simulink model "modeloLineales"  (R2022a)
settings: Solver=VariableStepAuto  StartTime=0.0  StopTime=300  FixedStep=6  RelTol=1e-3
model workspace (MAT data in the model file):
  ca = 0.001
  cb = 0.001
  ea = 0.001
  eb = 0.001
  pa = 2
  pb = 2
  u = 0.001
  v = 3
settings Model: Creator=Asus  LastModifiedBy=Abelino
settings DataIOCC: SaveFormat=Array  OutputTimes=tout

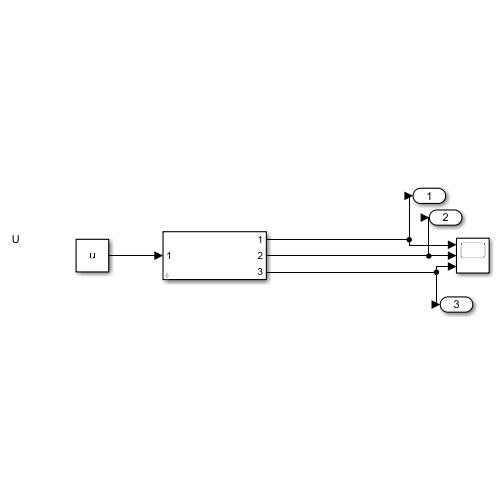
[thumbnail: Simulink's stored preview of the top-level diagram]
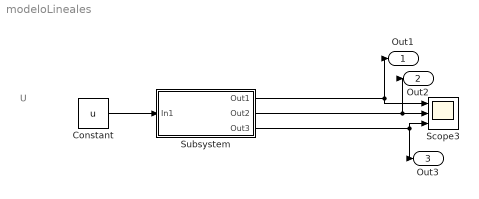
== system modeloLineales ==
  note: U
  Constant : Constant  Value=u
  Scope3 : Scope  NumInputPorts=3
  Subsystem : Subsystem  mask{ea=ea, eb=eb, ca=ca, cb=cb, pa=pa, pb=pb, v=v}
      mask prompts: ea "Tasa de extinción competidor A"; eb "Tasa de extinción del competidor B"; ca "Tasa de colonización del competidor A"; cb "Tasa de colonización del competidor B"; pa "Condición inicial x1"; pb "Condicion inicial x2"; v "Condicion inicial x3"
  Out1 : Outport
  Out2 : Outport  Port=2
  Out3 : Outport  Port=3
  wires:
  Subsystem/2(Out2) -> Out2/1, Scope3/2
  Subsystem/3(Out3) -> Scope3/3, Out3/1
  Subsystem/1(Out1) -> Scope3/1, Out1/1
  Constant/1 -> Subsystem/1(In1)

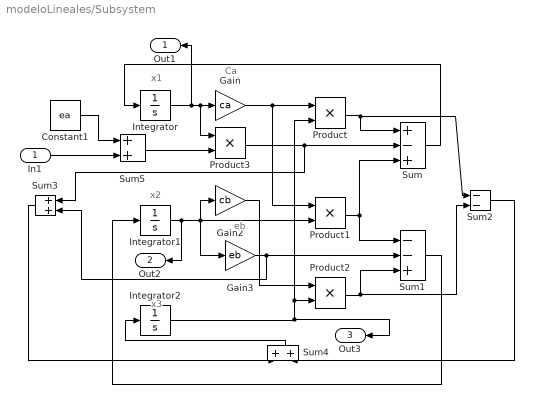
== system modeloLineales/Subsystem ==
  note: x1
  note: x3
  note: x2
  note: eb
  note: Ca
  In1 : Inport
  Constant1 : Constant  Value=ea
  Gain : Gain  Gain=ca
  Gain2 : Gain  Gain=cb
  Gain3 : Gain  Gain=eb
  Integrator : Integrator  InitialCondition=pa  LimitOutput=on  LowerSaturationLimit=0
  Integrator1 : Integrator  InitialCondition=pb  LimitOutput=on  LowerSaturationLimit=0
  Integrator2 : Integrator  InitialCondition=v  LimitOutput=on  LowerSaturationLimit=0
  Product{,1..3} (4 alike) : Product
  Sum : Sum  Inputs=+-+
  Sum1 : Sum  Inputs=--+
  Sum2 : Sum  Inputs=--
  Sum3 : Sum
  Sum4 : Sum
  Sum5 : Sum
  Out1 : Outport
  Out2 : Outport  Port=2
  Out3 : Outport  Port=3
  wires:
  Integrator/1 -> Out1/1, Product3/1, Gain/1
  Gain/1 -> Product1/1, Product/1
  Integrator2/1 -> Product/2, Product2/2, Out3/1
  Sum4/1 -> Integrator2/1
  Product2/1 -> Sum2/2, Sum1/3
  Sum2/1 -> Sum4/2
  Product/1 -> Sum2/1, Sum/1
  Gain2/1 -> Product2/1
  Gain3/1 -> Sum3/2, Sum1/2
  Sum3/1 -> Sum4/1
  Integrator1/1 -> Out2/1, Gain3/1, Gain2/1, Product1/2
  Sum/1 -> Integrator/1
  Product1/1 -> Sum/3, Sum1/1
  Sum1/1 -> Integrator1/1
  Constant1/1 -> Sum5/1
  In1/1 -> Sum5/2
  Sum5/1 -> Product3/2
  Product3/1 -> Sum3/1, Sum/2
